simulink model "Copy_of_Constant_vel"  (R2024b)
settings: Solver=FixedStepAuto  StartTime=0.0  StopTime=10  FixedStep=0.001  RelTol=1e-3
libraries: simulink x3
settings Model: Creator=cpero  LastModifiedBy=cpero

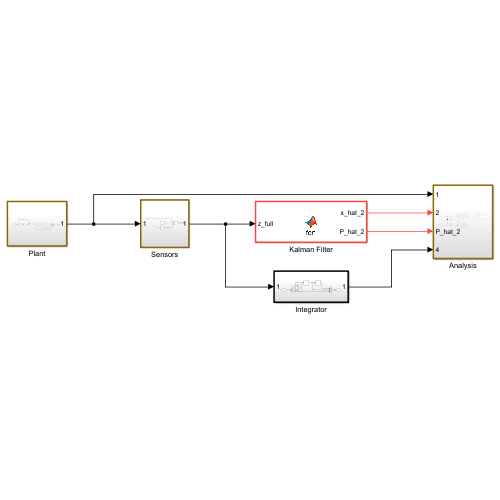
[thumbnail: Simulink's stored preview of the top-level diagram]
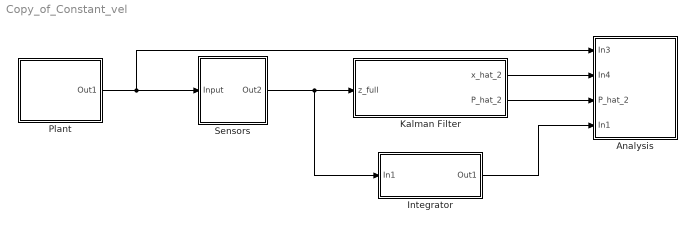
== system Copy_of_Constant_vel ==
  Analysis : Subsystem
  Integrator : Subsystem
  Kalman Filter : MATLAB Function  TreatAsAtomicUnit=on
  Plant : Subsystem
  Sensors : Subsystem
  wires:
  Plant/1(Out1) -> Analysis/1(In3), Sensors/1(Input)
  Sensors/1(Out2) -> Integrator/1(In1), Kalman Filter/1(z_full)
  Kalman Filter/1(x_hat_2) -> Analysis/2(In4)
  Integrator/1(Out1) -> Analysis/4(In1)
  Kalman Filter/2(P_hat_2) -> Analysis/3(P_hat_2)

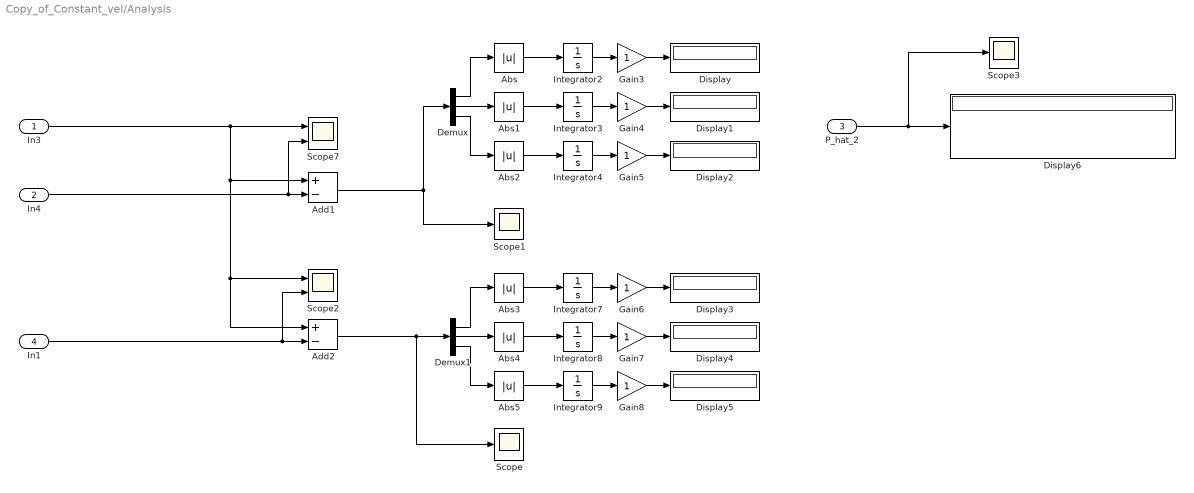
== system Copy_of_Constant_vel/Analysis ==
  In3 : Inport
  In4 : Inport  Port=2
  P_hat_2 : Inport  Port=3
  In1 : Inport  Port=4
  Abs{,1..5} (6 alike) : Abs  SaturateOnIntegerOverflow=off
  Add1 : Sum  Inputs=+-
  Add2 : Sum  Inputs=+-
  Demux : Demux  Outputs=3
  Demux1 : Demux  Outputs=3
  Display{,1..6} (7 alike) : Display
  Gain{3..8} (6 alike) : Gain
  Integrator{2..4,7..9} (6 alike) : Integrator
  Scope : Scope
  Scope1 : Scope
  Scope2 : Scope  NumInputPorts=2
  Scope3 : Scope
  Scope7 : Scope  NumInputPorts=2
  wires:
  Gain5/1 -> Display2/1
  Abs/1 -> Integrator2/1
  Abs4/1 -> Integrator8/1
  Add1/1 -> Demux/1, Scope1/1
  Demux/1 -> Abs/1
  Demux1/2 -> Abs4/1
  Abs1/1 -> Integrator3/1
  Demux/2 -> Abs1/1
  Gain3/1 -> Display/1
  Gain8/1 -> Display5/1
  In4/1 -> Scope7/2, Add1/2
  Integrator3/1 -> Gain4/1
  Abs2/1 -> Integrator4/1
  Abs3/1 -> Integrator7/1
  Integrator2/1 -> Gain3/1
  Demux/3 -> Abs2/1
  Gain4/1 -> Display1/1
  Integrator4/1 -> Gain5/1
  Gain7/1 -> Display4/1
  Integrator9/1 -> Gain8/1
  Integrator7/1 -> Gain6/1
  Integrator8/1 -> Gain7/1
  Gain6/1 -> Display3/1
  Demux1/3 -> Abs5/1
  Abs5/1 -> Integrator9/1
  Demux1/1 -> Abs3/1
  In1/1 -> Scope2/2, Add2/2
  Add2/1 -> Scope/1, Demux1/1
  P_hat_2/1 -> Scope3/1, Display6/1
  In3/1 -> Add2/1, Scope2/1, Add1/1, Scope7/1

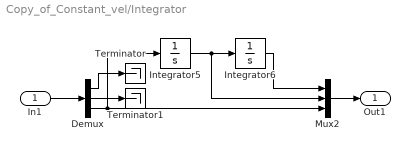
== system Copy_of_Constant_vel/Integrator ==
  In1 : Inport
  Demux : Demux  Outputs=3
  Integrator5 : Integrator
  Integrator6 : Integrator
  Mux2 : Mux  Inputs=3
  Terminator : Terminator
  Terminator1 : Terminator
  Out1 : Outport
  wires:
  Integrator5/1 -> Integrator6/1, Mux2/2
  Demux/3 -> Mux2/3, Integrator5/1
  Integrator6/1 -> Mux2/1
  Mux2/1 -> Out1/1
  In1/1 -> Demux/1
  Demux/1 -> Terminator/1
  Demux/2 -> Terminator1/1

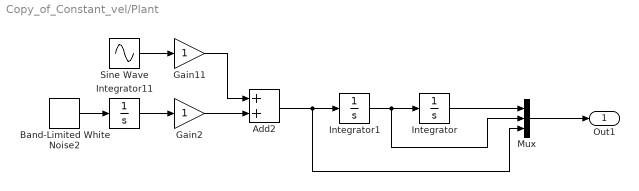
== system Copy_of_Constant_vel/Plant ==
  Add2 : Sum
  Band-Limited White Noise2 : simulink/Sources/Band-Limited White Noise  Cov=[1e-3]  Ts=0.001  seed=[4]
  Gain11 : Gain
  Gain2 : Gain
  Integrator : Integrator
  Integrator1 : Integrator
  Integrator11 : Integrator
  Mux : Mux  Inputs=3
  Sine Wave : Sin  SampleTime=0
  Out1 : Outport
  wires:
  Integrator1/1 -> Mux/2, Integrator/1
  Add2/1 -> Mux/3, Integrator1/1
  Gain2/1 -> Add2/2
  Gain11/1 -> Add2/1
  Sine Wave/1 -> Gain11/1
  Band-Limited White Noise2/1 -> Integrator11/1
  Integrator11/1 -> Gain2/1
  Integrator/1 -> Mux/1
  Mux/1 -> Out1/1

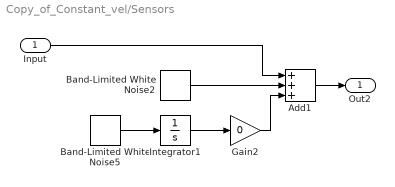
== system Copy_of_Constant_vel/Sensors ==
  Input : Inport
  Add1 : Sum  Inputs=+++
  Band-Limited White Noise2 : simulink/Sources/Band-Limited White Noise  Cov=[1e-3; 1e-9; 1e-5]  Ts=1e-3  seed=[1 2 3]
  Band-Limited White Noise5 : simulink/Sources/Band-Limited White Noise  Cov=[1e-3; 0; 1e-5]  Ts=1e-3  seed=[4 5 6]
  Gain2 : Gain  Gain=0
  Integrator1 : Integrator
  Out2 : Outport
  wires:
  Input/1 -> Add1/1
  Band-Limited White Noise2/1 -> Add1/2
  Band-Limited White Noise5/1 -> Integrator1/1
  Integrator1/1 -> Gain2/1
  Gain2/1 -> Add1/3
  Add1/1 -> Out2/1

== matlab function Copy_of_Constant_vel/Kalman Filter ==
  settings: updateMethod=DISCRETE
  data: z_full input; x_hat_2 output; P_hat_2 output
function [x_hat_2, P_hat_2] = fcn(z_full)

persistent x_hat_2_prior P_hat_2_prior i

dt = 1e-3;

F = [1 dt 0.5*dt^2;
     0 1 dt
     0 0 1];
H_full = eye(3);

q = 1; % Process noise strength
Q = q * [dt^4/4, dt^3/2, dt^2/2; 
          dt^3/2, dt^2,   dt;    
          dt^2/2, dt,     1];
R_full = diag([100, 1, 50]);

if isempty(x_hat_2_prior)
    x_hat_2_prior = [0;0;0];
    P_hat_2_prior = 0.02*eye(3);
    i=0;
end

%Predict
x_hat_1 = F*x_hat_2_prior;
P_hat_1 = F*P_hat_2_prior*F' + Q;

sensor_vec = [0; 0; 1];
if mod(i,70) == 0
    sensor_vec(1) = 1;
end
if mod(i,10) == 0
    sensor_vec(2) = 1;
end

if ~isequal(sensor_vec, [0; 0; 1]) 
    %Update
    sensor_indicies = sensor_vec==1;
    num_sensors = length(sensor_indicies);
    H = H_full(sensor_indicies,:);
    R = R_full(sensor_indicies,sensor_indicies);
    z = z_full(sensor_indicies);

    y = z - H*x_hat_1;
    S = H*P_hat_1*H' + R;
    K = P_hat_1*H'*inv(S);
    x_hat_2 = x_hat_1 + K*y;
    P_hat_2 = (eye(num_sensors) - K*H)*P_hat_1;
else
    x_hat_2 = x_hat_1;
    P_hat_2 = P_hat_1;
end

x_hat_2_prior = x_hat_2;
P_hat_2_prior = P_hat_2;
i = i+1;
